simulink model "G24i_fixed_load"  (R2014a)
settings: Solver=ode45  StartTime=0.0  StopTime=10.0  RelTol=1e-3
values from neighbouring files (symbols this model uses):
  ArrayCurrent = [1.05303e-05 0.0329007487024 0.0659314357778 0.100205 0.132978217474 0.166891516648 0.200872978445 0.234107600227 0.267513340222 0.302009988541 0.336322 0.36979130469 ... (44440 elements, 101x440)]    [ArrayCurrent.mat]    (also in Genrate_SC_mod.m = fitresult_normal_g42(V,G); temp3.m = fitresult(V,G))
  ArrayVoltage = [0 0.01 0.02 0.03 0.04 0.05 0.06 0.07 0.08 0.09 0.1 0.11 ... (440 elements, 1x440)]    [ArrayVoltage.mat]    (also in Genrate_SC_mod.m = (0:0.01:max(Voltage)); temp3.m = (0:0.01:max(Voltage)))
  Irradiance = (min(Lux):50:max(Lux))    [Genrate_SC_mod.m]    (also in Irradiance.mat = [0 50 100 150 200 250 300 350 400 450 500 550 ... (101 eleme; temp3.m)
libraries: fl_lib x5, nesl_utility x4, simulink_extras x1
settings Model: Creator=kartik.karuna  LastModifiedBy=kartik.karuna

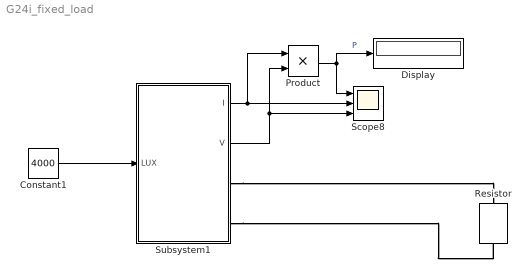
== system G24i_fixed_load ==
  Constant1 : Constant  Value=4000
  Display : Display
  Product : Product  RndMeth=Zero
  Resistor : fl_lib/Electrical/Electrical Elements/Resistor  R=4 Ohm  i_specify=off  i_priority=High  i=0 A  v_specify=off  v_priority=High  v=0 V
  Scope8 : Scope  NumInputPorts=3
      settings: YMin=-15000~2.53676~-7500  YMax=15000~2.53681~7500  SaveName=ScopeData9
  Subsystem1 : Subsystem
  wires:
  Product/1 -> Display/1, Scope8/1  "P"
  Subsystem1/2(V) -> Product/2, Scope8/3
  Subsystem1/1(I) -> Product/1, Scope8/2
  Constant1/1 -> Subsystem1/1(LUX)
  connections:
  Subsystem1/RConn2 -- Resistor/RConn1
  Subsystem1/RConn1 -- Resistor/LConn1

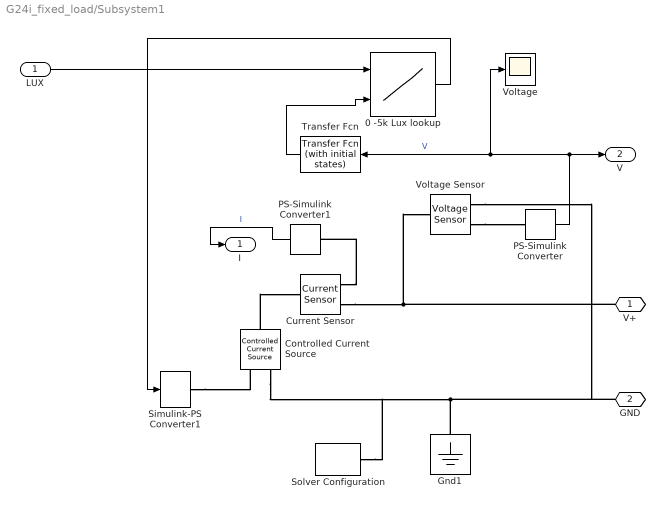
== system G24i_fixed_load/Subsystem1 ==
  LUX : Inport
  0 -5k Lux lookup : Lookup_n-D  BreakpointsForDimension1=Irradiance  BreakpointsForDimension2=ArrayVoltage  Table=ArrayCurrent  RndMeth=Simplest  InputSameDT=on
  Controlled Current Source : fl_lib/Electrical/Electrical Sources/Controlled Current Source
  Current Sensor : fl_lib/Electrical/Electrical Sensors/Current Sensor
  Gnd1 : fl_lib/Electrical/Electrical Elements/Electrical Reference
  PS-Simulink Converter : nesl_utility/PS-Simulink Converter  PhysicalDomain=network_engine_domain  SubClassName=ps_output  LeftPortType=input  RightPortType=output  PseudoPeriodic=off  Frequencies=[]  Unit=1  AffineConversion=off
  PS-Simulink Converter1 : nesl_utility/PS-Simulink Converter  PhysicalDomain=network_engine_domain  SubClassName=ps_output  LeftPortType=input  RightPortType=output  PseudoPeriodic=off  Frequencies=[]  Unit=1  AffineConversion=off
  Simulink-PS Converter1 : nesl_utility/Simulink-PS Converter  PhysicalDomain=network_engine_domain  SubClassName=ps_input  LeftPortType=input  RightPortType=output  PseudoPeriodic=off  Frequencies=[]  NoiseDistribution=none  NoiseParameters=[]  Unit=1  AffineConversion=off  InputFiltering=off  SimscapeFilterOrder=1  InputFilterTimeConstant=0.001  UdotUserProvided=1
  Solver Configuration : nesl_utility/Solver Configuration  PhysicalDomain=network_engine_domain  SubClassName=solver  LeftPortType=input  RightPortType=generic  Accelerate=off  Tones=[]  Harmonics=[]  SimulateNoise=off  Profile=off  UseLocalSampling=off  EnableSwitchedLinearOptims=on  FrequencyDomain=off  UseCCode=off  RelTol=0.001  AbsTol=1e-06  MinStep=1e-09  ToWorkspace=off  DoDC=off  ResidualTolerance=1e-09  UseLocalSolver=off  LocalSolverChoice=NE_BACKWARD_EULER_ADVANCER  LocalSolverSampleTime=0.001  DoFixedCost=off  MaxNonlinIter=3  MaxModeIter=2  LinearAlgebra=Sparse  DelaysMemoryBudget=1024  AutomaticFiltering=on  FilteringTimeConstant=0.001
  Transfer Fcn : simulink_extras/Additional Linear/Transfer Fcn (with initial states)  N=[1]  D="[.0001  1]"  X0=0
  Voltage : Scope
      settings: YMin=0.815936  YMax=0.815936  SaveName=ScopeData6
  Voltage Sensor : fl_lib/Electrical/Electrical Sensors/Voltage Sensor
  V+ : PMIOPort  Port=1  Side=Right
  GND : PMIOPort  Port=2  Side=Right
  I : Outport
  V : Outport  Port=2
  wires:
  0 -5k Lux lookup/1 -> Simulink-PS Converter1/1
  LUX/1 -> 0 -5k Lux lookup/1
  Transfer Fcn/1 -> 0 -5k Lux lookup/2
  PS-Simulink Converter/1 -> V/1, Transfer Fcn/1, Voltage/1  "V"
  PS-Simulink Converter1/1 -> I/1  "I"
  connections:
  Voltage Sensor/RConn1 -- PS-Simulink Converter/LConn1
  Current Sensor/RConn1 -- PS-Simulink Converter1/LConn1
  Controlled Current Source/LConn1 -- Current Sensor/LConn1
  Simulink-PS Converter1/RConn1 -- Controlled Current Source/RConn1
  Current Sensor/RConn2 -- V+/RConn1 -- Voltage Sensor/LConn1
  Gnd1/LConn1 -- Controlled Current Source/RConn2 -- Solver Configuration/RConn1 -- GND/RConn1 -- Voltage Sensor/RConn2
